simulink model "dynamics"  (R2023b)
settings: Solver=ode8  StartTime=0.0  StopTime=2000  FixedStep=.1  RelTol=1e-3
values from neighbouring files (symbols this model uses):
  ic = string_config2(p)    [main.m]
undefined symbols (not defined in the file or in its folder): p
settings Model: Creator=cyrus  LastModifiedBy=cyrus

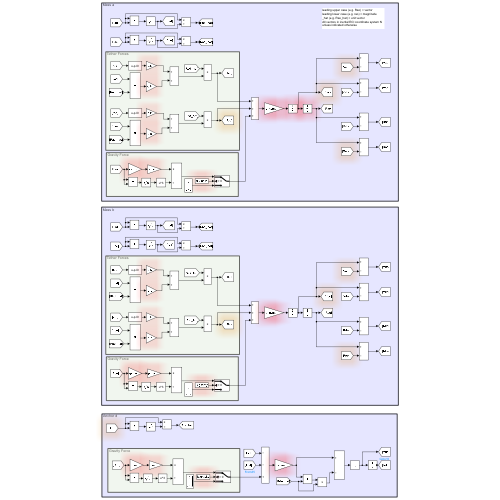
[thumbnail: Simulink's stored preview of the top-level diagram]
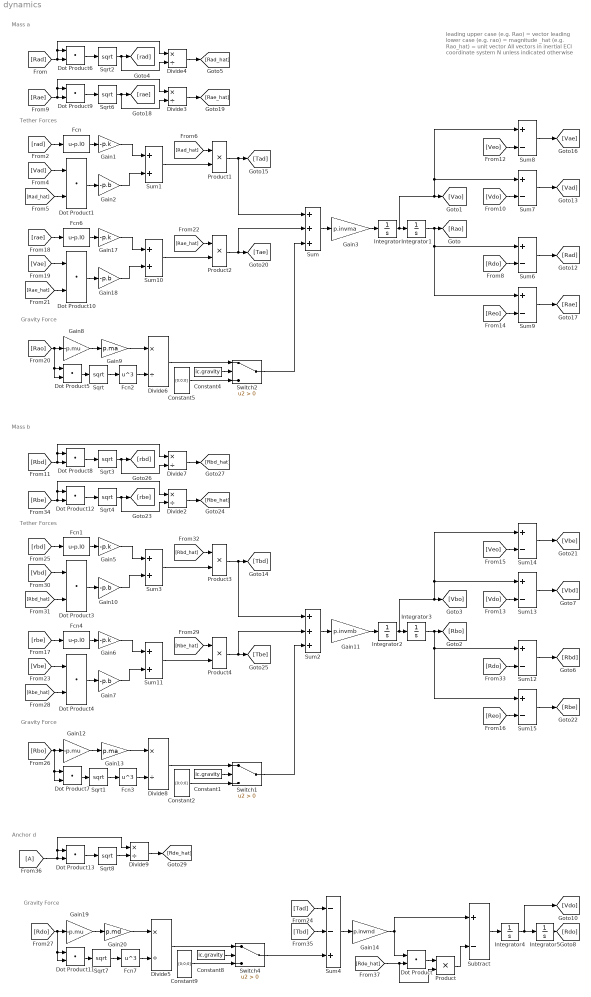
== system dynamics ==
  note: Gravity Force
  note: Anchor d
  note: Tether Forces
  note: leading upper case (e.g. Rao) = vector
      | leading lower case (e.g. rao) = magnitude
      | _hat (e.g. Rao_hat) = unit vector
      | All vectors in inertial ECI coordinate system N unless indicated otherwise
  note: Mass a
  note: Gravity Force
  note: Gravity Force
  note: Tether Forces
  note: Mass b
  Constant1 : Constant  Value=ic.gravity
  Constant2 : Constant  Value=[0;0;0]  VectorParams1D=off
  Constant4 : Constant  Value=ic.gravity
  Constant5 : Constant  Value=[0;0;0]  VectorParams1D=off
  Constant8 : Constant  Value=ic.gravity
  Constant9 : Constant  Value=[0;0;0]  VectorParams1D=off
  Divide{2..9} (8 alike) : Product  Inputs=*/
  Dot Product{,1,3..13} (13 alike) : DotProduct  OutDataTypeStr=Inherit: Inherit via internal rule
  Fcn{,1,4,6} (4 alike) : Fcn  Expr=u-p.l0
  Fcn2 : Fcn  Expr=u^3
  Fcn3 : Fcn  Expr=u^3
  Fcn7 : Fcn  Expr=u^3
  From36 : From
  Gain{1,5..6,17} (4 alike) : Gain  Gain=-p.k
  Gain{2,7,10,18} (4 alike) : Gain  Gain=-p.b
  Gain11 : Gain  Gain=p.invmb
  Gain12 : Gain  Gain=-p.mu
  Gain13 : Gain  Gain=p.ma
  Gain14 : Gain  Gain=p.invmd
  Gain19 : Gain  Gain=-p.mu
  Gain20 : Gain  Gain=p.md
  Gain3 : Gain  Gain=p.invma
  Gain8 : Gain  Gain=-p.mu
  Gain9 : Gain  Gain=p.ma
  Integrator : Integrator  InitialCondition=ic.NVao0
  Integrator1 : Integrator  InitialCondition=ic.NRao0
  Integrator{2..5} (4 alike) : Integrator
  Product{,1..4} (5 alike) : Product
  Sqrt{,1..4,6..8} (8 alike) : Sqrt
  Subtract : Sum  Inputs=+-
  Sum : Sum  Inputs=+++
  Sum{1,3,10..11} (4 alike) : Sum
  Sum{6..9,12..15} (8 alike) : Sum  Inputs=+-
  Sum2 : Sum  Inputs=+++
  Sum4 : Sum  Inputs=--+
  Switch1 : Switch  Criteria=u2 > Threshold  SaturateOnIntegerOverflow=off  InputSameDT=off
  Switch2 : Switch  Criteria=u2 > Threshold  SaturateOnIntegerOverflow=off  InputSameDT=off
  Switch4 : Switch  Criteria=u2 > Threshold  SaturateOnIntegerOverflow=off  InputSameDT=off
  wires:
  [Rad] -> Divide4/1, Dot Product6/1, Dot Product6/2
  Dot Product6/1 -> Sqrt2/1
  Sqrt2/1 -> Divide4/2, [rad]
  Divide4/1 -> [Rad_hat]
  [rad] -> Fcn/1
  Fcn/1 -> Gain1/1
  Gain1/1 -> Sum1/1
  [Vad] -> Dot Product1/1
  [Rad_hat] -> Dot Product1/2
  Dot Product1/1 -> Gain2/1
  Gain2/1 -> Sum1/2
  Sum1/1 -> Product1/2
  Sum/1 -> Gain3/1
  Gain3/1 -> Integrator/1
  Integrator/1 -> Integrator1/1, Sum7/1, Sum8/1, [Vao]
  Integrator1/1 -> Sum9/1, Sum6/1, [Rao]
  [Rao] -> Dot Product5/2, Dot Product5/1, Gain8/1
  Gain8/1 -> Gain9/1
  Gain9/1 -> Divide6/1
  Fcn2/1 -> Divide6/2
  Sqrt/1 -> Fcn2/1
  Dot Product5/1 -> Sqrt/1
  Integrator4/1 -> [Vdo], Integrator5/1
  Sum4/1 -> Gain14/1
  Integrator5/1 -> [Rdo]
  Product1/1 -> Sum/1, [Tad]
  Constant4/1 -> Switch2/2
  Constant5/1 -> Switch2/3
  Divide6/1 -> Switch2/1
  [Rdo] -> Sum6/2
  Sum6/1 -> [Rad]
  Sum7/1 -> [Vad]
  [Vdo] -> Sum7/2
  [Veo] -> Sum8/2
  Sum8/1 -> [Vae]
  Sum9/1 -> [Rae]
  [Reo] -> Sum9/2
  Dot Product9/1 -> Sqrt6/1
  Sqrt6/1 -> Divide3/2, [rae]
  Divide3/1 -> [Rae_hat]
  [Rae] -> Divide3/1, Dot Product9/1, Dot Product9/2
  [Rad_hat] -> Product1/1
  Fcn6/1 -> Gain17/1
  [Vae] -> Dot Product10/1
  Product2/1 -> Sum/2, [Tae]
  Dot Product10/1 -> Gain18/1
  Gain17/1 -> Sum10/1
  Gain18/1 -> Sum10/2
  Sum10/1 -> Product2/2
  [rae] -> Fcn6/1
  [Rae_hat] -> Dot Product10/2
  [Rae_hat] -> Product2/1
  Switch2/1 -> Sum/3
  [Rdo] -> Dot Product11/2, Dot Product11/1, Gain19/1
  Divide5/1 -> Switch4/1
  Constant8/1 -> Switch4/2
  Constant9/1 -> Switch4/3
  Dot Product11/1 -> Sqrt7/1
  Gain19/1 -> Gain20/1
  Sqrt7/1 -> Fcn7/1
  Gain20/1 -> Divide5/1
  Fcn7/1 -> Divide5/2
  [Reo] -> Sum15/2
  Sum15/1 -> [Rbe]
  Switch1/1 -> Sum2/3
  [Rbe_hat] -> Dot Product4/2
  Sum11/1 -> Product4/2
  [rbe] -> Fcn4/1
  Product4/1 -> Sum2/2, [Tbe]
  Gain6/1 -> Sum11/1
  Gain7/1 -> Sum11/2
  Fcn4/1 -> Gain6/1
  [Vbe] -> Dot Product4/1
  Dot Product4/1 -> Gain7/1
  [Rdo] -> Sum12/2
  Sqrt4/1 -> Divide2/2, [rbe]
  [Rbe_hat] -> Product4/1
  [Vdo] -> Sum13/2
  Sum13/1 -> [Vbd]
  Sum14/1 -> [Vbe]
  Dot Product12/1 -> Sqrt4/1
  [Veo] -> Sum14/2
  Fcn1/1 -> Gain5/1
  [Rbo] -> Dot Product7/2, Dot Product7/1, Gain12/1
  Divide2/1 -> [Rbe_hat]
  [Rbd_hat] -> Product3/1
  Divide8/1 -> Switch1/1
  Sum2/1 -> Gain11/1
  Constant1/1 -> Switch1/2
  Constant2/1 -> Switch1/3
  Sum3/1 -> Product3/2
  [Vbd] -> Dot Product3/1
  Fcn3/1 -> Divide8/2
  Dot Product8/1 -> Sqrt3/1
  Gain12/1 -> Gain13/1
  Sqrt1/1 -> Fcn3/1
  Gain13/1 -> Divide8/1
  Integrator3/1 -> Sum15/1, Sum12/1, [Rbo]
  Gain10/1 -> Sum3/2
  Dot Product3/1 -> Gain10/1
  Product3/1 -> Sum2/1, [Tbd]
  Gain5/1 -> Sum3/1
  [Rbe] -> Divide2/1, Dot Product12/1, Dot Product12/2
  [Rbd_hat] -> Dot Product3/2
  [rbd] -> Fcn1/1
  Sqrt3/1 -> Divide7/2, [rbd]
  Gain11/1 -> Integrator2/1
  Sum12/1 -> [Rbd]
  Divide7/1 -> [Rbd_hat]
  Integrator2/1 -> Integrator3/1, Sum13/1, Sum14/1, [Vbo]
  Dot Product7/1 -> Sqrt1/1
  [Rbd] -> Divide7/1, Dot Product8/1, Dot Product8/2
  [Tad] -> Sum4/1
  [Tbd] -> Sum4/2
  Switch4/1 -> Sum4/3
  Sqrt8/1 -> Divide9/2
  Divide9/1 -> [Rde_hat]
  From36/1 -> Divide9/1, Dot Product13/1, Dot Product13/2
  Dot Product13/1 -> Sqrt8/1
  Gain14/1 -> Dot Product/1, Subtract/1
  [Rde_hat] -> Product/2, Dot Product/2
  Dot Product/1 -> Product/1
  Product/1 -> Subtract/2
  Subtract/1 -> Integrator4/1
